simulink model "HDLSS"  (R2024a)
settings: Solver=FixedStepDiscrete  StartTime=0.0  StopTime=stopTime  RelTol=1e-3
undefined symbols (not defined in the file or in its folder): CONST
libraries: HDL_ieee_8021513 x3, dspsrcs4 x2
settings Model: DataTypeOverride=Off  Creator=cotti  LastModifiedBy=cotti
settings OptimizationCC: BlockReduction=off  ConditionallyExecuteInputs=off  DefaultParameterBehavior=Inlined  InheritOutputTypeSmallerThanSingle=on
settings DebuggingCC: ArtificialAlgebraicLoopMsg=error  SingleTaskRateTransMsg=error
settings HardwareCC: ProdBitPerPointer=32  ProdBitPerSizeT=32  ProdBitPerPtrDiffT=32  ProdLargestAtomicFloat=None  ProdIntDivRoundTo=Undefined  ProdEndianess=Unspecified  ProdWordSize=32  ProdHWDeviceType=ASIC/FPGA->ASIC/FPGA  TargetBitPerLong=64  TargetBitPerPointer=64  TargetBitPerSizeT=64  TargetBitPerPtrDiffT=64  TargetLongLongMode=on  TargetIntDivRoundTo=Zero  TargetEndianess=LittleEndian  TargetWordSize=64  TargetHWDeviceType=Custom Processor->MATLAB Host Computer  ProdEqTarget=off

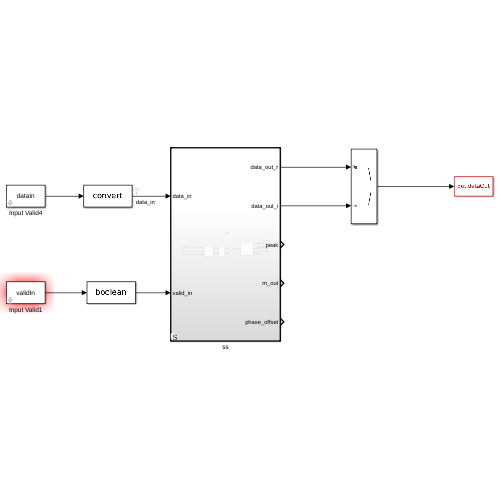
[thumbnail: Simulink's stored preview of the top-level diagram]
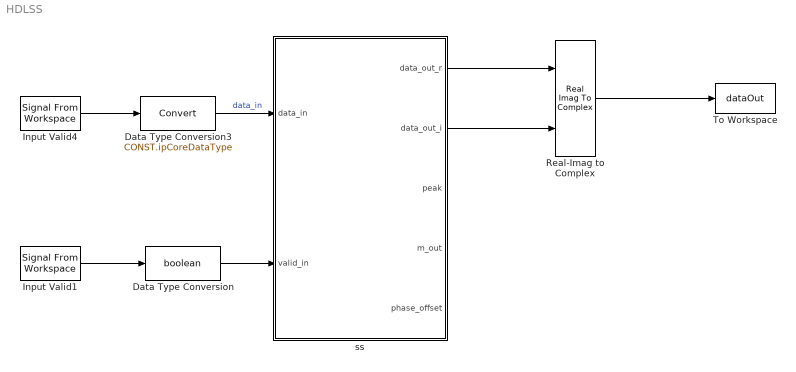
== system HDLSS ==
  Data Type Conversion : DataTypeConversion  OutDataTypeStr=boolean  SaturateOnIntegerOverflow=off  RndMeth=Floor
  Data Type Conversion3 : DataTypeConversion  OutDataTypeStr=CONST.ipCoreDataType  SaturateOnIntegerOverflow=off  RndMeth=Floor
  Input Valid1 : dspsrcs4/Signal From Workspace  X=validIn  Ts=1/CONST.fADC  nsamps=1  OutputAfterFinalValue=Setting to zero  ignoreOrWarnInputAndFrameLengths=off  OutputFrames=off
  Input Valid4 : dspsrcs4/Signal From Workspace  X=dataIn  Ts=1/CONST.fADC  nsamps=1  OutputAfterFinalValue=Setting to zero  ignoreOrWarnInputAndFrameLengths=off  OutputFrames=off
  Real-Imag to Complex : RealImagToComplex
  To Workspace : ToWorkspace  VariableName=dataOut  SampleTime=1/CONST.fPHY
      settings: Save2DSignal=2-D array (concatenate along first dimension)
  ss : Subsystem
  wires:
  Input Valid4/1 -> Data Type Conversion3/1
  Input Valid1/1 -> Data Type Conversion/1
  Data Type Conversion3/1 -> ss/1(data_in)  "data_in"
  Data Type Conversion/1 -> ss/2(valid_in)
  ss/2(data_out_i) -> Real-Imag to Complex/2
  ss/1(data_out_r) -> Real-Imag to Complex/1
  Real-Imag to Complex/1 -> To Workspace/1

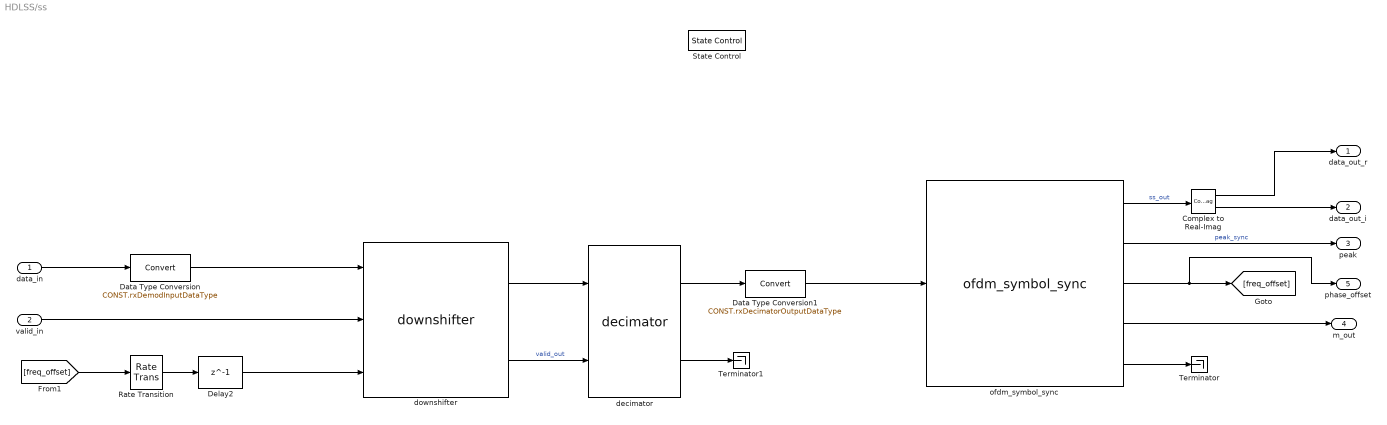
== system HDLSS/ss ==
  data_in : Inport
  valid_in : Inport  Port=2
  Complex to Real-Imag : ComplexToRealImag
  Data Type Conversion : DataTypeConversion  OutDataTypeStr=CONST.rxDemodInputDataType  SaturateOnIntegerOverflow=off  RndMeth=Floor
  Data Type Conversion1 : DataTypeConversion  OutDataTypeStr=CONST.rxDecimatorOutputDataType  SaturateOnIntegerOverflow=off  RndMeth=Floor
  Delay2 : Delay  DelayLength=1  InitialCondition=0  UseCircularBuffer=on
  Rate Transition : RateTransition  OutPortSampleTime=1/CONST.fDAC
  State Control : StateControl  StateControl=Synchronous
  Terminator : Terminator
  Terminator1 : Terminator
  decimator : HDL_ieee_8021513/decimator  SystemSampleTime=-1  VariantActivationTime=update diagram  AllowFlexibleInterface=on  Latency=0  AutoFrameSizeCalculation=off
      settings: SourceProductName=HDL IEEE 8021513
  downshifter : HDL_ieee_8021513/downshifter  SystemSampleTime=-1  VariantActivationTime=update diagram  AllowFlexibleInterface=on  Latency=0  AutoFrameSizeCalculation=off
      settings: SourceProductName=HDL IEEE 8021513
  ofdm_symbol_sync : HDL_ieee_8021513/ofdm_symbol_sync  SystemSampleTime=-1  VariantActivationTime=update diagram  AllowFlexibleInterface=on  Latency=0  AutoFrameSizeCalculation=off
      settings: SourceProductName=HDL IEEE 8021513
  data_out_r : Outport  VectorParamsAs1DForOutWhenUnconnected=off
  data_out_i : Outport  Port=2  VectorParamsAs1DForOutWhenUnconnected=off
  peak : Outport  Port=3  VectorParamsAs1DForOutWhenUnconnected=off
  m_out : Outport  Port=4  VectorParamsAs1DForOutWhenUnconnected=off
  phase_offset : Outport  Port=5  VectorParamsAs1DForOutWhenUnconnected=off
  wires:
  [freq_offset] -> Rate Transition/1
  valid_in/1 -> downshifter/2
  ofdm_symbol_sync/5 -> Terminator/1
  ofdm_symbol_sync/3 -> phase_offset/1, [freq_offset]
  Data Type Conversion1/1 -> ofdm_symbol_sync/1
  data_in/1 -> Data Type Conversion/1
  Rate Transition/1 -> Delay2/1
  Delay2/1 -> downshifter/3
  decimator/2 -> Terminator1/1
  ofdm_symbol_sync/2 -> peak/1  "peak_sync"
  decimator/1 -> Data Type Conversion1/1
  downshifter/1 -> decimator/1
  Data Type Conversion/1 -> downshifter/1
  downshifter/2 -> decimator/2  "valid_out"
  ofdm_symbol_sync/4 -> m_out/1
  ofdm_symbol_sync/1 -> Complex to Real-Imag/1  "ss_out"
  Complex to Real-Imag/1 -> data_out_r/1
  Complex to Real-Imag/2 -> data_out_i/1
